simulink model "PH1_full_simp"  (R2017a)
settings: Solver=ode23s  StartTime=0.0  StopTime=.2  MaxStep=1e-6  RelTol=1e-3
libraries: powerlib x28
settings Model: Creator=erich  LastModifiedBy=Administrador

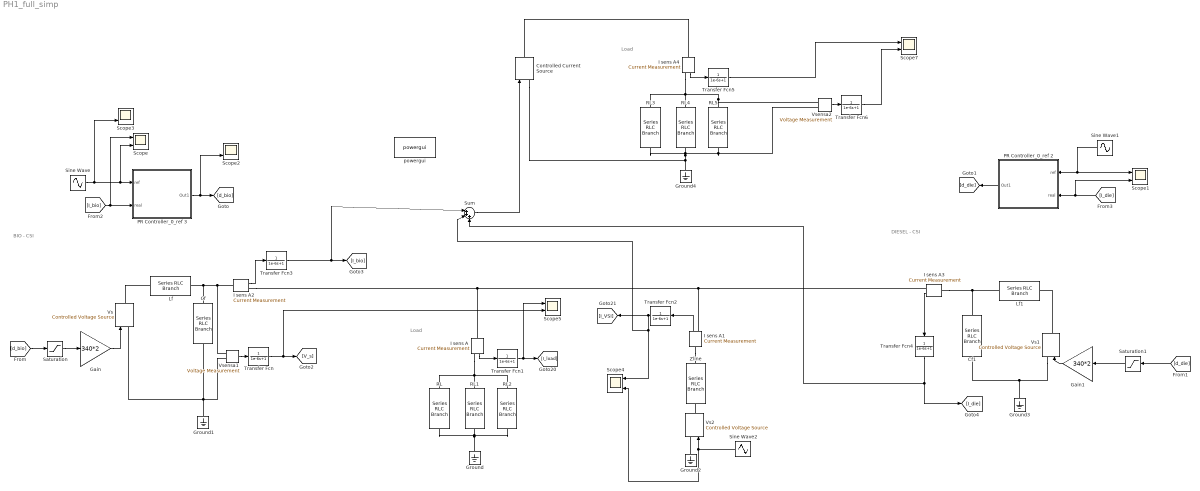
== system PH1_full_simp ==
  note: BIO - CSI
  note: Load
  note: DIESEL - CSI
  note: Load
  Cf : powerlib/Elements/Series RLC Branch  LConnTagsString=__new0  RConnTagsString=__new0  BranchType=C  Resistance=1  Inductance=1e-3  SetiL0=off  InitialCurrent=0  Capacitance=22e-6  Setx0=off  InitialVoltage=0  Measurements=None
  Cf1 : powerlib/Elements/Series RLC Branch  LConnTagsString=__new0  RConnTagsString=__new0  BranchType=C  Resistance=1  Inductance=1e-3  SetiL0=off  InitialCurrent=0  Capacitance=22e-6  Setx0=off  InitialVoltage=0  Measurements=None
  Controlled Current Source : powerlib/Electrical Sources/Controlled Current Source  Initialize=on  Source_Type=AC  Amplitude=0  Phase=0  Frequency=0  Measurements=None
  Gain : Gain  Gain=340*2
  Gain1 : Gain  Gain=340*2
  Ground{,1..4} (5 alike) : powerlib/Elements/Ground  LConnTagsString=a
  I sens A{,1..4} (5 alike) : powerlib/Measurements/Current Measurement  PhasorSimulation=off  OutputType=Complex  PSBequivalent=0
  Lf : powerlib/Elements/Series RLC Branch  LConnTagsString=__new0  RConnTagsString=__new0  BranchType=RL  Resistance=.1  Inductance=40e-3  SetiL0=off  InitialCurrent=0  Capacitance=1e-6  Setx0=off  InitialVoltage=0  Measurements=None
  Lf1 : powerlib/Elements/Series RLC Branch  LConnTagsString=__new0  RConnTagsString=__new0  BranchType=RL  Resistance=.1  Inductance=30e-3  SetiL0=off  InitialCurrent=0  Capacitance=1e-6  Setx0=off  InitialVoltage=0  Measurements=None
  PR Controller_0_ref 2 : Subsystem  mask{Kp=40/100, Ki=200, wa=2, w0=60*2*pi, st_time=0}
      mask prompts: Kp "Ganancia Proporcional"; Ki "Ganancia Integral"; wa "Ancho camapana resonancia"; w0 "Frecuencia Central"; st_time "Tiempo muerto (Start)"
      mask Display:
      | port_label('input',1,'ref')
      | port_label('input',2,'sens')
      | port_label('output',1,'out')
      | 
      | plot(.4+[0:.01:pi/10], .32+sin(40*[0:.01:pi/10])/13)
      | 
      | plot([.4 .6],.05+[.5 .7])
      | plot([.4 .6],.05+[.9 .7])
      | plot([.4 .4],.05+[.9 .5])
      | 
      | text(.27,.37,'\fontsize{25} \int', 'texmode', 'on')
  PR Controller_0_ref 3 : Subsystem  mask{Kp=40/100, Ki=200, wa=2, w0=60*2*pi, st_time=0}
      mask prompts: Kp "Ganancia Proporcional"; Ki "Ganancia Integral"; wa "Ancho camapana resonancia"; w0 "Frecuencia Central"; st_time "Tiempo muerto (Start)"
      mask Display:
      | port_label('input',1,'ref')
      | port_label('input',2,'sens')
      | port_label('output',1,'out')
      | 
      | plot(.4+[0:.01:pi/10], .32+sin(40*[0:.01:pi/10])/13)
      | 
      | plot([.4 .6],.05+[.5 .7])
      | plot([.4 .6],.05+[.9 .7])
      | plot([.4 .4],.05+[.9 .5])
      | 
      | text(.27,.37,'\fontsize{25} \int', 'texmode', 'on')
  RL : powerlib/Elements/Series RLC Branch  LConnTagsString=__new0  RConnTagsString=__new0  BranchType=R  Resistance=10  Inductance=500e-3  SetiL0=off  InitialCurrent=0  Capacitance=100e-6  Setx0=off  InitialVoltage=0  Measurements=None
  RL1 : powerlib/Elements/Series RLC Branch  LConnTagsString=__new0  RConnTagsString=__new0  BranchType=RL  Resistance=10  Inductance=5.2  SetiL0=off  InitialCurrent=0  Capacitance=100e-6  Setx0=off  InitialVoltage=0  Measurements=None
  RL2 : powerlib/Elements/Series RLC Branch  LConnTagsString=__new0  RConnTagsString=__new0  BranchType=C  Resistance=30  Inductance=500e-3  SetiL0=off  InitialCurrent=0  Capacitance=2000e-6  Setx0=off  InitialVoltage=0  Measurements=None
  RL3 : powerlib/Elements/Series RLC Branch  LConnTagsString=__new0  RConnTagsString=__new0  BranchType=R  Resistance=10  Inductance=500e-3  SetiL0=off  InitialCurrent=0  Capacitance=100e-6  Setx0=off  InitialVoltage=0  Measurements=None
  RL4 : powerlib/Elements/Series RLC Branch  LConnTagsString=__new0  RConnTagsString=__new0  BranchType=RL  Resistance=10  Inductance=5.2  SetiL0=off  InitialCurrent=0  Capacitance=100e-6  Setx0=off  InitialVoltage=0  Measurements=None
  RL5 : powerlib/Elements/Series RLC Branch  LConnTagsString=__new0  RConnTagsString=__new0  BranchType=C  Resistance=30  Inductance=500e-3  SetiL0=off  InitialCurrent=0  Capacitance=2000e-6  Setx0=off  InitialVoltage=0  Measurements=None
  Saturation : Saturate  UpperLimit=.5  LowerLimit=-.5
  Saturation1 : Saturate  UpperLimit=.5  LowerLimit=-.5
  Scope{,1..5,7} (7 alike) : Scope  NumInputPorts=2
  Sine Wave : Sin  Amplitude=10  Frequency=2*pi*60  SampleTime=0
  Sine Wave1 : Sin  Amplitude=10  Frequency=2*pi*60  SampleTime=0
  Sine Wave2 : Sin  Amplitude=170  Frequency=2*pi*60  SampleTime=0
  Sum : Sum  Inputs=|+++
  Transfer Fcn{,1..6} (7 alike) : TransferFcn  Denominator=[1e-6 1]
  Vs : powerlib/Electrical Sources/Controlled Voltage Source  Initialize=on  Source_Type=AC  Amplitude=0  Phase=0  Frequency=0  Measurements=None
  Vs1 : powerlib/Electrical Sources/Controlled Voltage Source  Initialize=on  Source_Type=AC  Amplitude=0  Phase=0  Frequency=0  Measurements=None
  Vs2 : powerlib/Electrical Sources/Controlled Voltage Source  Initialize=on  Source_Type=AC  Amplitude=0  Phase=0  Frequency=0  Measurements=None
  Vsensa1 : powerlib/Measurements/Voltage Measurement  PhasorSimulation=off  OutputType=Complex  PSBequivalent=0
  Vsensa2 : powerlib/Measurements/Voltage Measurement  PhasorSimulation=off  OutputType=Complex  PSBequivalent=0
  Zline : powerlib/Elements/Series RLC Branch  LConnTagsString=__new0  RConnTagsString=__new0  BranchType=RL  Resistance=.001  Inductance=10e-6  SetiL0=off  InitialCurrent=0  Capacitance=100e-6  Setx0=off  InitialVoltage=0  Measurements=None
  powergui : powerlib/powergui  Priority=1  SimulationMode=Continuous  SampleTime=50e-6  frequency=60  Iterations=50  frequencyindice=0  Pbase=100e6  ErrMax=1e-4  UnitsV=kV  UnitsW=MW  buscounter=0  FunctionMessages=off  echomessages=off  EnableUseOfTLC=off  CurrentSourceSwitches=off  DisableSnubberDevices=off  DisableRonSwitches=off  DisableVfSwitches=off  DisplayEquations=off  SolverType=Tustin/Backward Euler (TBE)  Interpol=off  ExternalGateDelay=off  methode=off  Ts=100  x0status=blocks  SPID=on  SwTol=0  HookPort=off  RestoreLinks=warning  ResistiveCurrentMeasurement=off  Frange=[0:2:500]  Ylog=off  Xlog=on  ShowGrid=off  save=off  variable=ZData  structure=0  ZoomFFT=off  StartTime=0.0  cycles=1  DisplayStyle=1  fundamental=60  FreqAxis=off  MaxFrequency=1000  frequencyindicesteady=1  RmsSteady=1  display=off
  wires:
  Gain1/1 -> Vs1/1
  Gain/1 -> Vs/1
  I sens A/1 -> Transfer Fcn1/1
  PR Controller_0_ref 3/1(Out1) -> Scope2/2, [d_bio]
  [d_bio] -> Saturation/1
  PR Controller_0_ref 2/1(Out1) -> [d_die]
  [d_die] -> Saturation1/1
  [I_bio] -> Scope/1, PR Controller_0_ref 3/2(real)
  Sine Wave/1 -> Scope3/2, PR Controller_0_ref 3/1(ref), Scope/2
  Transfer Fcn/1 -> Scope5/2, [V_s]
  Vsensa1/1 -> Transfer Fcn/1
  Transfer Fcn1/1 -> Scope5/1, [I_load]
  Transfer Fcn2/1 -> [I_VSI], Sum/2, Scope4/1
  Transfer Fcn3/1 -> Sum/1, [I_bio]
  [I_die] -> Scope1/2, PR Controller_0_ref 2/2(real)
  Sine Wave1/1 -> Scope1/1, PR Controller_0_ref 2/1(ref)
  Saturation/1 -> Gain/1
  Saturation1/1 -> Gain1/1
  I sens A3/1 -> Transfer Fcn4/1
  I sens A2/1 -> Transfer Fcn3/1
  Sine Wave2/1 -> Scope4/2, Vs2/1
  I sens A1/1 -> Transfer Fcn2/1
  Transfer Fcn4/1 -> Sum/3, [I_die]
  Sum/1 -> Controlled Current Source/1
  I sens A4/1 -> Transfer Fcn5/1
  Transfer Fcn5/1 -> Scope7/1
  Vsensa2/1 -> Transfer Fcn6/1
  Transfer Fcn6/1 -> Scope7/2
  connections:
  Vs1/LConn1 -- Cf1/RConn1 -- Ground3/LConn1
  Vs1/RConn1 -- Lf1/LConn1
  Lf1/RConn1 -- I sens A3/LConn1 -- Cf1/LConn1
  Vs/LConn1 -- Ground1/LConn1 -- Cf/RConn1 -- Vsensa1/LConn2
  Vs/RConn1 -- Lf/LConn1
  RL1/LConn1 -- RL/LConn1 -- I sens A/RConn1 -- RL2/LConn1
  RL/RConn1 -- RL2/RConn1 -- Ground/LConn1 -- RL1/RConn1
  Vs2/RConn1 -- Zline/RConn1
  Ground2/LConn1 -- Vs2/LConn1
  Vsensa1/LConn1 -- I sens A2/LConn1 -- Cf/LConn1 -- Lf/RConn1
  I sens A2/RConn1 -- I sens A3/RConn1 -- I sens A1/RConn1 -- I sens A/LConn1
  I sens A1/LConn1 -- Zline/LConn1
  RL3/RConn1 -- Vsensa2/LConn2 -- RL5/RConn1 -- Controlled Current Source/LConn1 -- Ground4/LConn1 -- RL4/RConn1
  RL5/LConn1 -- RL4/LConn1 -- RL3/LConn1 -- I sens A4/RConn1 -- Vsensa2/LConn1
  Controlled Current Source/RConn1 -- I sens A4/LConn1

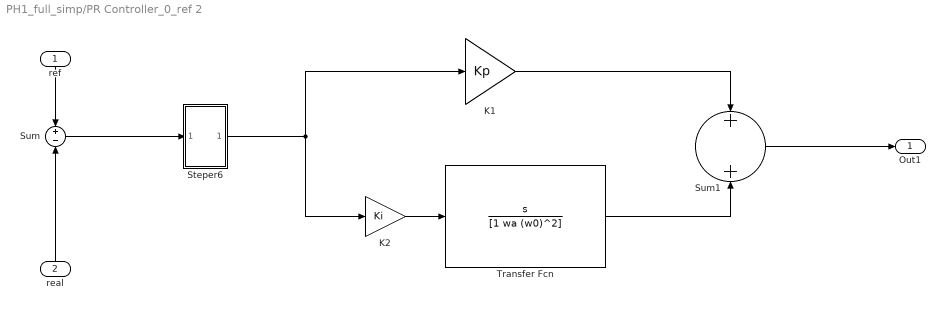
== system PH1_full_simp/PR Controller_0_ref 2 ==
  ref : Inport
  real : Inport  Port=2
  K1 : Gain  Gain=Kp
  K2 : Gain  Gain=Ki
  Steper6 : Subsystem
  Sum : Sum  Inputs=+-
  Sum1 : Sum  Inputs=+|+
  Transfer Fcn : TransferFcn  Numerator=[1 0]  Denominator=[1 wa (w0)^2]
  Out1 : Outport
  wires:
  real/1 -> Sum/2
  ref/1 -> Sum/1
  Sum/1 -> Steper6/1(In1)
  K1/1 -> Sum1/1
  Transfer Fcn/1 -> Sum1/2
  K2/1 -> Transfer Fcn/1
  Steper6/1(Out1) -> K1/1, K2/1
  Sum1/1 -> Out1/1

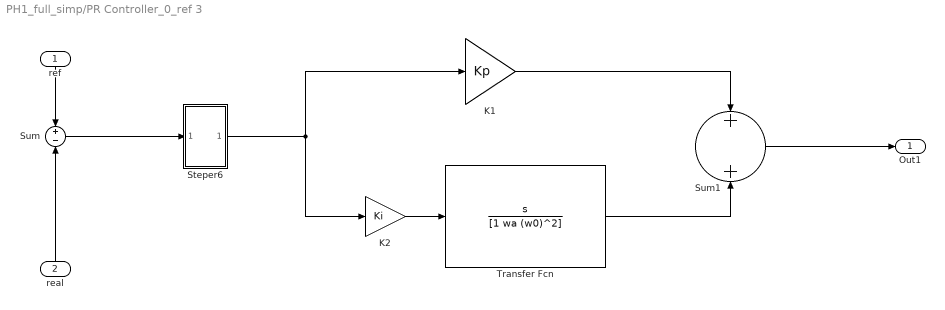
== system PH1_full_simp/PR Controller_0_ref 3 ==
  ref : Inport
  real : Inport  Port=2
  K1 : Gain  Gain=Kp
  K2 : Gain  Gain=Ki
  Steper6 : Subsystem
  Sum : Sum  Inputs=+-
  Sum1 : Sum  Inputs=+|+
  Transfer Fcn : TransferFcn  Numerator=[1 0]  Denominator=[1 wa (w0)^2]
  Out1 : Outport
  wires:
  real/1 -> Sum/2
  ref/1 -> Sum/1
  Sum/1 -> Steper6/1(In1)
  K1/1 -> Sum1/1
  Transfer Fcn/1 -> Sum1/2
  K2/1 -> Transfer Fcn/1
  Steper6/1(Out1) -> K1/1, K2/1
  Sum1/1 -> Out1/1

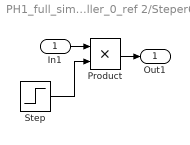
== system PH1_full_simp/PR Controller_0_ref 2/Steper6 ==
  In1 : Inport
  Product : Product
  Step : Step  Time=st_time  SampleTime=0
  Out1 : Outport
  wires:
  Product/1 -> Out1/1
  In1/1 -> Product/1
  Step/1 -> Product/2

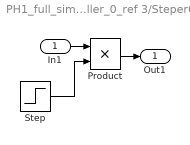
== system PH1_full_simp/PR Controller_0_ref 3/Steper6 ==
  In1 : Inport
  Product : Product
  Step : Step  Time=st_time  SampleTime=0
  Out1 : Outport
  wires:
  Product/1 -> Out1/1
  In1/1 -> Product/1
  Step/1 -> Product/2
